simulink model "Problem_4"  (R2020a)
settings: Solver=VariableStepAuto  StartTime=0.0  StopTime=10.0  RelTol=1e-3
settings Model: Creator=Admin  LastModifiedBy=Admin

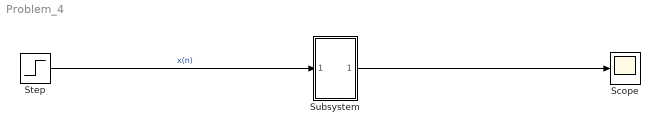
== system Problem_4 ==
  Scope : Scope
  Step : Step  SampleTime=0
  Subsystem : Subsystem
  wires:
  Step/1 -> Subsystem/1(x(n))  "x(n)"
  Subsystem/1(y(n)) -> Scope/1

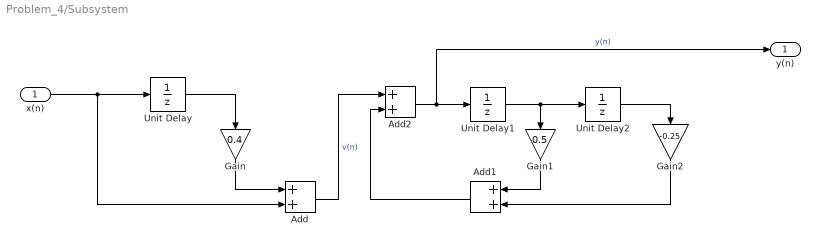
== system Problem_4/Subsystem ==
  x(n) : Inport
  Add : Sum
  Add1 : Sum
  Add2 : Sum
  Gain : Gain  Gain=0.4
  Gain1 : Gain  Gain=0.5
  Gain2 : Gain  Gain=-0.25
  Unit Delay : UnitDelay  SampleTime=-1  HasFrameUpgradeWarning=on
  Unit Delay1 : UnitDelay  SampleTime=-1  HasFrameUpgradeWarning=on
  Unit Delay2 : UnitDelay  SampleTime=-1  HasFrameUpgradeWarning=on
  y(n) : Outport
  wires:
  Gain/1 -> Add/1
  x(n)/1 -> Unit Delay/1, Add/2
  Unit Delay/1 -> Gain/1
  Unit Delay2/1 -> Gain2/1
  Gain1/1 -> Add1/1
  Add2/1 -> y(n)/1, Unit Delay1/1  "y(n)"
  Gain2/1 -> Add1/2
  Unit Delay1/1 -> Gain1/1, Unit Delay2/1
  Add/1 -> Add2/1  "v(n)"
  Add1/1 -> Add2/2
